simulink model "MOD_Hbridge_Ctrl"  (R2018b)
settings: Solver=VariableStepDiscrete  StartTime=0  StopTime=30  RelTol=1e-3
PreLoadFcn:
  | if(exist('MBDS_ModelCallback', 'file'))
  |    MBDS_ModelCallback('PreLoad');
  | end
PostLoadFcn:
  | if(exist('MBDS_ModelCallback', 'file'))
  |    MBDS_ModelCallback('PostLoad');
  | end
InitFcn:
  | if(exist('MBDS_ModelCallback', 'file'))
  |    MBDS_ModelCallback('Init');
  | end
StartFcn:
  | if(exist('MBDS_ModelCallback', 'file'))
  |    MBDS_ModelCallback('Start');
  | end
StopFcn:
  | if(exist('MBDS_ModelCallback', 'file'))
  |    MBDS_ModelCallback('Stop');
  | end
undefined symbols (not defined in the file): sigbuilder_block
libraries: simulink x1
(part 2 of 2)

== stateflow chart MOD_Hbridge_Ctrl/Model/MOD_Hbridge_Ctrl_/FullHBridgeCtrl ==
  state H_SimulationMode
    en:
    u8_HBridgeSts= u8_HSimu;
    i8_HB1SideCtrl = i8_HBOFF;
    i8_HB2SideCtrl = i8_HBOFF;
    bo_OpenLoadDetectCtrl=false;
    du:
    i8_HB1SideCtrl = i8_HB1SideSimuVal;
    i8_HB2SideCtrl = i8_HB2SideSimuVal;
    bo_OpenLoadDetectCtrl=bo_OpenLoadDetectSimuVal;
  state H_StandAlone
    state H_ForceBrake
      en:
      u16_Timer=uint16(1);
      u8_HBridgeSts= u8_HForceBrake;
      i8_HB1SideCtrl = i8_HBLS;
      i8_HB2SideCtrl = i8_HBLS;
      bo_OpenLoadDetectCtrl=false;
      du:
      u16_Timer++;
    state H_OFF
      en:
      u16_Timer=uint16(1);
      u8_HBridgeSts= u8_HOFF;
      i8_HB1SideCtrl = i8_HBOFF;
      i8_HB2SideCtrl = i8_HBOFF;
      bo_OpenLoadDetectCtrl=false;
      du:
      u16_Timer++;
    state H_Failure
      en:
      u8_HBridgeSts= u8_HFail;
      i8_HB1SideCtrl = i8_HBOFF;
      i8_HB2SideCtrl = i8_HBOFF;
      bo_OpenLoadDetectCtrl=false;
    state H_OLD
      en:
      u16_Timer=uint16(1);
      u8_HBridgeSts= u8_HOLD;
      i8_HB1SideCtrl = i8_HBLS;
      i8_HB2SideCtrl = i8_HBOFF;
      bo_OpenLoadDetectCtrl=true;
      du:
      u16_Timer++;
    state H_WaitForNoRqst
      en:
      u8_HBridgeSts= u8_HWait;
      i8_HB1SideCtrl = i8_HBOFF;
      i8_HB2SideCtrl = i8_HBOFF;
      bo_OpenLoadDetectCtrl=false;
    state H_Down
      en:
      u16_Timer=uint16(1);
      u8_HBridgeSts= u8_HDown;
      i8_HB1SideCtrl = i8_HBOFF;
      i8_HB2SideCtrl = i8_HBOFF;
      bo_OpenLoadDetectCtrl=false;
      du:
      i8_HB1SideCtrl = i8_HBLS;
      i8_HB2SideCtrl = i8_HBHS;
      u16_Timer++;
    state H_Up
      en:
      u16_Timer=uint16(1);
      u8_HBridgeSts= u8_HUp;
      i8_HB1SideCtrl = i8_HBOFF;
      i8_HB2SideCtrl = i8_HBOFF;
      bo_OpenLoadDetectCtrl=false;
      du:
      i8_HB1SideCtrl = i8_HBHS;
      i8_HB2SideCtrl = i8_HBLS;
      u16_Timer++;
    state H_Brake
      en:
      u16_Timer=uint16(1);
      u8_HBridgeSts= u8_HBrake;
      i8_HB1SideCtrl = i8_HBLS;
      i8_HB2SideCtrl = i8_HBLS;
      bo_OpenLoadDetectCtrl=false;
      du:
      u16_Timer++;
    (default) -> H_ForceBrake
    H_Failure -> H_OFF : /* Request to turn H bridge OFF*/
        | [bo_UpRqst == false && bo_DownRqst == false]
    H_ForceBrake -> H_WaitForNoRqst : [u16_Timer >= u16_BrakeTime]
    H_OFF -> H_OLD : /* Request to turn H bridge ON or OLD intervaltime*/
        | [bo_UpRqst == true ||...
        | bo_DownRqst == true ||...
        | u16_Timer >= u16_OpenLoadIntervalTime]
    H_OLD -> H_Failure [order 1] : /* Open Load Detected */
        | [u16_Timer >= u16_OpenLoadDetectTime&&...
        | (u16_HB1SideDiag!=uint16(0x0000)||...
        | u16_HB2SideDiag!=uint16(0x0000))]
    H_WaitForNoRqst -> H_OFF : /* Wait till no Request to avoid start
        | moving actuators after POR*/
        | [bo_UpRqst == false &&...
        | bo_DownRqst == false]
    H_OLD -> H_OFF [order 2] : /* No Request to turn H bridge ON*/
        | [bo_UpRqst == false &&...
        | bo_DownRqst == false&&...
        | u16_Timer >= u16_OpenLoadDetectTime]
    H_OLD -> H_Up [order 3] : /* Up Rqst - OLD not Detected */
        | [bo_UpRqst == true&&...
        | bo_DownRqst == false&&...
        | u16_Timer >= u16_OpenLoadDetectTime]
    H_OLD -> H_Down [order 4] : /* Down Rqst - OLD not Detected */
        | [bo_UpRqst == false&&...
        | bo_DownRqst == true&&...
        | u16_Timer >= u16_OpenLoadDetectTime]
    H_Up -> H_Brake : /* Up Not Rqst or Timeout or error */
        | [bo_UpRqst == false ||...
        | u16_HB1SideDiag!=uint16(0x0000)||...
        | u16_HB2SideDiag!=uint16(0x0000)||...
        | u16_Timer >= u16_MaxActivationTime]
    H_Brake -> H_Up [order 2] : /* Up Request after Brake*/
        | [bo_UpRqst == true&&...
        | bo_DownRqst == false&&...
        | u16_Timer >= u16_BrakeTime]
    H_Brake -> H_Down [order 3] : /* Down Request after Brake */
        | [bo_UpRqst == false&&...
        | bo_DownRqst == true&&...
        | u16_Timer >= u16_BrakeTime]
    H_Down -> H_Brake : /* Down Not Rqst or Timeout  or error*/
        | [bo_DownRqst == false ||...
        | u16_HB1SideDiag!=uint16(0x0000)||...
        | u16_HB2SideDiag!=uint16(0x0000)||...
        | u16_Timer >= u16_MaxActivationTime]
    H_Brake -> H_OFF [order 4] : /* Request to turn H bridge OFF  after Brake*/
        | [bo_UpRqst == false &&...
        |  bo_DownRqst == false &&...
        | u16_Timer >= u16_BrakeTime]
    H_Brake -> H_Failure [order 1] : /* Failure Detected after Brake */
        | [u16_Timer >= u16_BrakeTime&&...
        | (u16_HB1SideDiag!=uint16(0x0000)||...
        | u16_HB2SideDiag!=uint16(0x0000))]
  state H_SimulationBrake
    en:
    u16_Timer=uint16(1);
    u8_HBridgeSts= u8_HBrakeSimulation;
    i8_HB1SideCtrl = i8_HBLS;
    i8_HB2SideCtrl = i8_HBLS;
    bo_OpenLoadDetectCtrl=false;
    du:
    u16_Timer++;
  (default) -> H_SimulationMode
  H_SimulationMode -> H_StandAlone : [bo_WorkingMode==true]
  H_SimulationBrake -> H_SimulationMode : [u16_Timer >= u16_BrakeTime]
  H_StandAlone -> H_SimulationBrake : [bo_WorkingMode==false]
  data: bo_UpRqst input boolean; bo_DownRqst input boolean; i8_HB1SideCtrl output int8 =0; i8_HB2SideCtrl output int8 =0; u16_Timer local uint16 =0; u16_HB1SideDiag input uint16; u16_HB2SideDiag input uint16; u16_BrakeTime input uint16; bo_OpenLoadDetectCtrl output boolean =false; u16_OpenLoadDetectTime input uint16; u8_HBridgeSts output uint8 =0; i8_HBHS local int8 =1; i8_HBLS local int8 =-1; i8_HBOFF local int8 =0; u8_HOFF local uint8 =0; u8_HBrake local uint8 =1; u8_HOLD local uint8 =2; u8_HUp local uint8 =3; u8_HDown local uint8 =4; u8_HFail local uint8 =5; u16_MaxActivationTime input uint16; u16_OpenLoadIntervalTime input uint16; u8_HWait local uint8 =6; i8_HB1SideSimuVal input int8; i8_HB2SideSimuVal input int8; bo_OpenLoadDetectSimuVal input boolean; bo_WorkingMode input boolean; u8_HSimu local uint8 =7; u8_HForceBrake local uint8 =8; u8_HBrakeSimulation local uint8 =9
